simulink model "ex6_3"  (R2019b)
settings: Solver=VariableStepAuto  StartTime=0.0  StopTime=10.0  RelTol=1e-3
undefined symbols (not defined in the file or in its folder): k
settings Model: Creator=Russty  LastModifiedBy=TimRo
settings DataIOCC: ReturnWorkspaceOutputs=off
settings DebuggingCC: ArithmeticOperatorsInVariantConditions=warning
settings SFSimCC: CustomCodeUndefinedFunction=UseInterfaceOnly

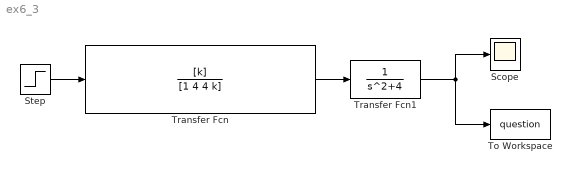
== system ex6_3 ==
  Scope : Scope
  Step : Step  Time=0  SampleTime=0.001
  To Workspace : ToWorkspace  VariableName=question  SaveFormat=Timeseries  SampleTime=-1
  Transfer Fcn : TransferFcn  Numerator=[k]  Denominator=[1 4 4 k]
  Transfer Fcn1 : TransferFcn  Denominator=[1 0 4]
  wires:
  Step/1 -> Transfer Fcn/1
  Transfer Fcn/1 -> Transfer Fcn1/1
  Transfer Fcn1/1 -> To Workspace/1, Scope/1
